simulink model "P4"  (R2020b)
settings: Solver=FixedStepDiscrete  StartTime=0.0  StopTime=20.0  RelTol=1e-3
settings Model: Creator=ASUS  LastModifiedBy=ASUS

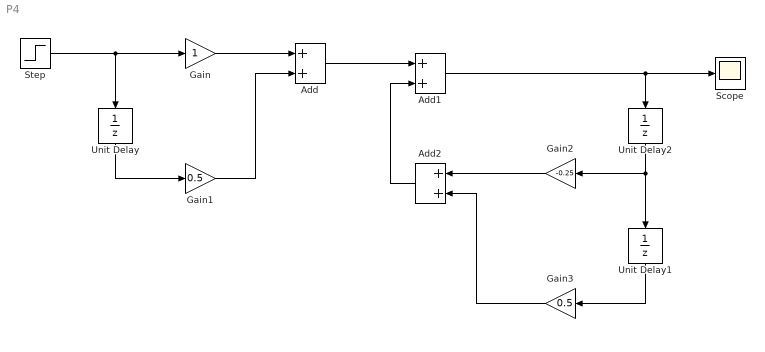
== system P4 ==
  Add : Sum
  Add1 : Sum
  Add2 : Sum
  Gain : Gain
  Gain1 : Gain  Gain=0.5
  Gain2 : Gain  Gain=-0.25
  Gain3 : Gain  Gain=0.5
  Scope : Scope
  Step : Step  SampleTime=0
  Unit Delay : UnitDelay  SampleTime=-1  HasFrameUpgradeWarning=on
  Unit Delay1 : UnitDelay  SampleTime=-1  HasFrameUpgradeWarning=on
  Unit Delay2 : UnitDelay  SampleTime=-1  HasFrameUpgradeWarning=on
  wires:
  Gain/1 -> Add/1
  Gain1/1 -> Add/2
  Add/1 -> Add1/1
  Add2/1 -> Add1/2
  Gain2/1 -> Add2/1
  Gain3/1 -> Add2/2
  Add1/1 -> Unit Delay2/1, Scope/1
  Step/1 -> Gain/1, Unit Delay/1
  Unit Delay2/1 -> Gain2/1, Unit Delay1/1
  Unit Delay1/1 -> Gain3/1
  Unit Delay/1 -> Gain1/1
